simulink model "lecture_sys"  (R2015a)
settings: Solver=ode3  StartTime=0.0  StopTime=10  FixedStep=.01  RelTol=1e-3
settings Model: Creator=lbremer  LastModifiedBy=lbremer

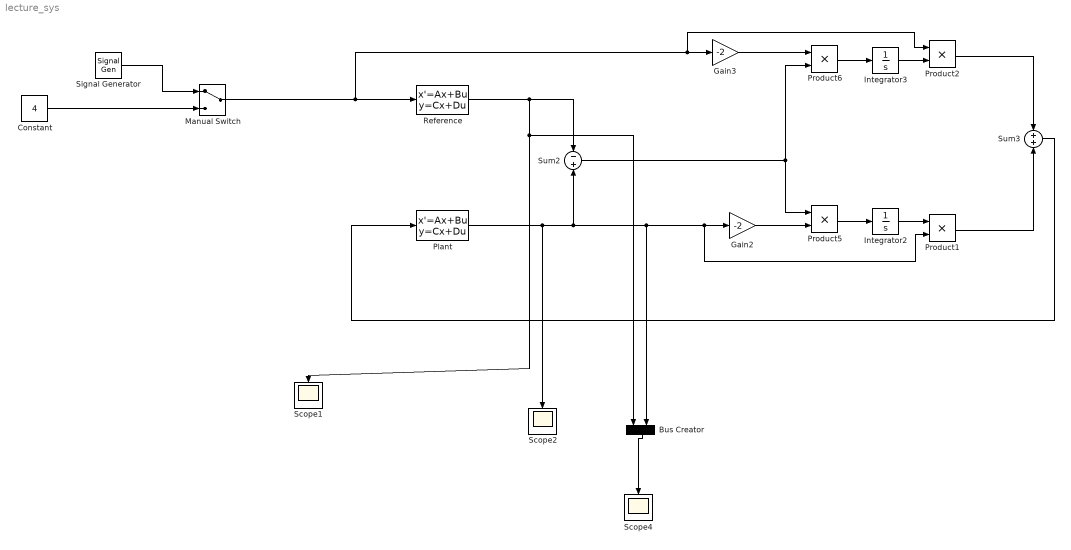
== system lecture_sys ==
  Bus Creator : BusCreator  Inputs=2
  Constant : Constant  Value=4
  Gain2 : Gain  Gain=-2
  Gain3 : Gain  Gain=-2
  Integrator2 : Integrator
  Integrator3 : Integrator
  Manual Switch : ManualSwitch
  "Plant " : StateSpace  B=3  D=0  X0=0
  Product{1..2,5..6} (4 alike) : Product
  "Reference " : StateSpace  A=-4  B=4  D=0  X0=0
  Scope1 : Scope
      settings: YMin=-1  YMax=1
  Scope2 : Scope
      settings: YMin=-1  YMax=1
  Scope4 : Scope
      settings: YMin=-1  YMax=1  SaveName=ScopeData4
  Signal Generator : SignalGenerator  Amplitude=4  Frequency=3  Units=rad/sec
  Sum2 : Sum  Inputs=-|+
  Sum3 : Sum  Inputs=+|+
  wires:
  "Reference "/1 -> Bus Creator/1, Scope1/1, Sum2/1
  Sum2/1 -> Product5/1, Product6/2
  Gain2/1 -> Product5/2
  Product5/1 -> Integrator2/1
  Gain3/1 -> Product6/1
  Product6/1 -> Integrator3/1
  Sum3/1 -> "Plant "/1
  Bus Creator/1 -> Scope4/1
  Constant/1 -> Manual Switch/2
  Signal Generator/1 -> Manual Switch/1
  Integrator2/1 -> Product1/1
  "Plant "/1 -> Product1/2, Gain2/1, Bus Creator/2, Sum2/2, Scope2/1
  Product1/1 -> Sum3/2
  Integrator3/1 -> Product2/2
  Manual Switch/1 -> Product2/1, Gain3/1, "Reference "/1
  Product2/1 -> Sum3/1
